simulink library "sm_flex_body_lib"  (R2016b)
settings: Solver=VariableStepAuto  StartTime=0.0  StopTime=10.0  RelTol=1e-3
values from neighbouring files (symbols this model uses):
  frameBody = splitBodyProps    [sm_flex_body_lib_fei_configure_beam.m]
undefined symbols (not defined in the file or in its folder): frameGraphic, X, Y, Z
undefined symbols (not defined in the file): beam_color, beam_opacity, beam_wall, beam_width, beamLink, brot_beamx, brot_beamy, brot_beamz, btra_beamx, elem_length, Extr_Data_Box, krot_beamx, krot_beamy, krot_beamz, ktra_beamx, rho, tau
libraries: sm_flex_body_lib x26, sm_lib x25, nesl_utility x24
(part 1 of 2)
Description:
  | Simscape Multibody Flexible Body Library v3.2
  | Copyright 2017 The MathWorks, Inc.
settings Model: Creator=smiller  LastModifiedBy=smiller

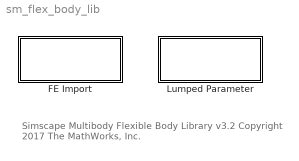
== system sm_flex_body_lib ==
  note: Simscape Multibody Flexible Body Library v3.2
      | Copyright 2017 The MathWorks, Inc.
  FE Import : Subsystem
  Lumped Parameter : Subsystem

== system sm_flex_body_lib/FE Import ==
  Bodies : Subsystem

== system sm_flex_body_lib/Lumped Parameter ==
  Bodies : Subsystem

== system sm_flex_body_lib/FE Import/Bodies ==
  Body 3 Frames : Subsystem  mask(Flexible Body via FE Import, 3 Frames){popup_massdistr=Per Interface Frame, mass=beamLink.iner.mass, com=beamLink.iner.com, moi=beamLink.iner.moi, poi=beamLink.iner.poi, splitBodyProps=beamLink.splitBodyProps(2).props, smallInertiaDim=1e-3, smallInertiaMass=1e-6, rigid_body_filename='BeamLink.stl', rigid_body_color=[0.0 0.4 0.6], rigid_body_opacity=0, intf_body_color=[0.0 0.4 0.6], intf_body_opacity=1, intf_graphic_color=[0.0 0.4 0.6], intf_graphic_opacity=0, rigidBodyFrame=2, T=beamLink.models(5).T, numframes=3, K=beamLink.models(5).K, M=beamLink.models(5).M, ksi=0.05, dofIdxMap=beamLink.models(5).dofIdxMap, tau=1e-6, H=beamLink.models(5).H, sensedFeaDofs_UI=[], numDynModes=20}
      mask prompts: popup_massdistr "Body Mass Distribution"; mass "Mass (kg)"; com "Center of Mass [xyz] (m)"; moi "Moments of Inertia (kg*m^2)"; poi "Products of Inertia (kg*m^2)"; splitBodyProps "Properties (structure)"; smallInertiaDim "Cube Side Length (m)"; smallInertiaMass "Cube Mass (kg)"; rigid_body_filename "Rigid Body File Name"; rigidBodyFrame "Rigid Body Frame"; T "Interface Frame Locations (m)"; K "Stiffness Matrix"; M "Mass Matrix"; ksi "Modal Damping Parameter"; dofIdxMap "Frame Dof Indices"; tau "Filter Time Constant (s)"; H "C-B Transformation Matrix"; sensedFeaDofs_UI "C-B Transformation Matrix Indices for Logging"
      mask help: Models a flexible body using a deflection model that relies on data imported from finite element software. Body deflection is superimposed on rigid body motion. The mass of the body can be assigned to the rigid body or distributed across each interface frame.
      mask init:
      | % Configure rigid and interface solids
      | [Nf, frameBody, frameGraphic] = sm_flex_body_lib_fei_configure_beam(gcb,splitBodyProps);
      | 
      | set_param(gcb,'numframes',num2str(Nf));
      | if(size(K,1)>0)
      |     set_param(gcb,'numDynModes',num2str(size(K,1)-Nf*6));
      | else
      |     set_param(gcb,'numDynModes','-');
      | end
      | 
      | % Sensed FEA dofs
      | if(isempty(sensedFeaDofs_UI))
      |     sensedFeaDofs = 1;
      | else
      |     sensedFeaDofs = sensedFeaDofs_UI;
      | end
      | 
      | % Create flexibility state-space model
      | [M2, L2, K2, H2] = sm_flex_body_lib_fei_form_def_matrices( ...
      |     H, M, K, ksi, Nf, dofIdxMap, rigidBodyFrame, sensedFeaDofs);
      | sys = sm_flex_body_lib_fei_form_statespace(Nf, M2, L2, K2, H2);
      | 
      | % Indices for Selector blocks at state-space output
      | sys_out_inds_frames = [1:Nf*6];
      | sys_out_width = length(sys_out_inds_frames)+length(sensedFeaDofs);
      | sys_out_inds_logging = [sys_out_width-length(sensedFeaDofs)+1:sys_out_width];
      settings: AttributesFormatString=|
      | Mass: %<popup_massdistr>
      | Interface Frames: %<numframes>
      | Rigid Frame: %<rigidBodyFrame>
      | # Dynamic Modes: %<numDynModes>
      mask Help: web('sm_flex_body_lib_fe_import_body.html');
      mask TypeOptions popup_massdistr: Single | Per Interface Frame
      mask Callback popup_massdistr:
      | maskObj = Simulink.Mask.get(gcb);
      | sms_h = maskObj.getDialogControl('cont_singlemass');
      | pms_h = maskObj.getDialogControl('cont_piecesmass');
      | int_h = maskObj.getDialogControl('cont_intfmass');
      | if strcmp(get_param(gcb,'popup_massdistr'),'Single')
      |     sms_h.Visible = 'on';
      |     int_h.Visible = 'on';
      |     pms_h.Visible = 'off';
      | else
      |     sms_h.Visible = 'off';
      |     int_h.Visible = 'off';
      |     pms_h.Visible = 'on';
      | end
      | clear maskObj sms_h pms_h int_h
      mask TypeOptions rigidBodyFrame: 1 | 2 | 3
      mask DialogControl cont_singlemass Prompt: Single Mass
      mask DialogControl cont_piecesmass Prompt: Body Mass Per Interface Frame
      mask DialogControl cont_intfmass Prompt: Interface Frame Minimum Mass
      mask DialogControl Control3 Prompt: Color [RGB]
      mask DialogControl Control4 Prompt: Opacity (0-1)
      mask DialogControl Control5 Prompt: Rigid Body Solid
      mask DialogControl Control6 Prompt: Interface Solid
      mask DialogControl Control7 Prompt: Interface Graphic
      mask Display: image('sm_flex_body_lib_feibeam3fr_IMAGE.png')
  Body 5 Frames : Subsystem  mask(Flexible Beam via FE Import, 5 Frames){popup_massdistr=Per Interface Frame, mass=beamLink.iner.mass, com=beamLink.iner.com, moi=beamLink.iner.moi, poi=beamLink.iner.poi, splitBodyProps=beamLink.splitBodyProps(3).props, smallInertiaDim=1e-3, smallInertiaMass=1e-6, rigid_body_filename='BeamLink.stl', rigid_body_color=[0.0 0.4 0.6], rigid_body_opacity=0, intf_body_color=[0.0 0.4 0.6], intf_body_opacity=1, intf_graphic_color=[0.0 0.4 0.6], intf_graphic_opacity=0, rigidBodyFrame=3, T=beamLink.models(7).T, numframes=5, K=beamLink.models(7).K, M=beamLink.models(7).M, ksi=0.05, dofIdxMap=beamLink.models(7).dofIdxMap, tau=1e-6, H=beamLink.models(7).H, sensedFeaDofs_UI=[], numDynModes=20}
      mask prompts: popup_massdistr "Body Mass Distribution"; mass "Mass (kg)"; com "Center of Mass [xyz] (m)"; moi "Moments of Inertia (kg*m^2)"; poi "Products of Inertia (kg*m^2)"; splitBodyProps "Properties (structure)"; smallInertiaDim "Cube Side Length (m)"; smallInertiaMass "Cube Mass (kg)"; rigid_body_filename "Rigid Body File Name"; rigidBodyFrame "Rigid Body Frame"; T "Interface Frame Locations (m)"; K "Stiffness Matrix"; M "Mass Matrix"; ksi "Modal Damping Parameter"; dofIdxMap "Frame Dof Indices"; tau "Filter Time Constant (s)"; H "C-B Transformation Matrix"; sensedFeaDofs_UI "C-B Transformation Matrix Indices for Logging"
      mask help: Models a flexible body using a deflection model that relies on data imported from finite element software. Body deflection is superimposed on rigid body motion. The mass of the body can be assigned to the rigid body or distributed across each interface frame.
      mask init: same as sm_flex_body_lib/FE Import/Bodies/Body 3 Frames
      settings: AttributesFormatString=|
      | Mass: %<popup_massdistr>
      | Interface Frames: %<numframes>
      | Rigid Frame: %<rigidBodyFrame>
      | # Dynamic Modes: %<numDynModes>
      mask Help: web('sm_flex_body_lib_fe_import_body.html');
      mask TypeOptions popup_massdistr: Single | Per Interface Frame
      mask Callback popup_massdistr:
      | maskObj = Simulink.Mask.get(gcb);
      | sms_h = maskObj.getDialogControl('cont_singlemass');
      | pms_h = maskObj.getDialogControl('cont_piecesmass');
      | int_h = maskObj.getDialogControl('cont_intfmass');
      | if strcmp(get_param(gcb,'popup_massdistr'),'Single')
      |     sms_h.Visible = 'on';
      |     int_h.Visible = 'on';
      |     pms_h.Visible = 'off';
      | else
      |     sms_h.Visible = 'off';
      |     int_h.Visible = 'off';
      |     pms_h.Visible = 'on';
      | end
      | clear maskObj sms_h pms_h int_h
      mask TypeOptions rigidBodyFrame: 1 | 2 | 3 | 4 | 5
      mask DialogControl cont_singlemass Prompt: Single Mass
      mask DialogControl cont_piecesmass Prompt: Body Mass Per Interface Frame
      mask DialogControl cont_intfmass Prompt: Interface Frame Minimum Mass
      mask DialogControl Control3 Prompt: Color [RGB]
      mask DialogControl Control4 Prompt: Opacity (0-1)
      mask DialogControl Control5 Prompt: Rigid Body Solid
      mask DialogControl Control6 Prompt: Interface Solid
      mask DialogControl Control7 Prompt: Interface Graphic
      mask Display: image('sm_flex_body_lib_feibeam5fr_IMAGE.png')
  Frame 1 : Subsystem  Variant=on  VariantControl=Variant1  OverrideUsingVariant=Flex
      settings: AttributesFormatString=%<ActiveVariant>
      mask Display:
      | blk = find_system(gcbh, 'SearchDepth', 1,'FollowLinks','on','LookUnderMasks','all', 'Parent', gcb, 'VariantObject', get_param(gcb,'activevariant'));
      | eval(get_param(blk, 'MaskDisplay'));
  Inertia F1 : Subsystem  mask(Flexibe Beam Frame Inertia and Graphic){frameSolid_elem=0, frameGraphic_elem=0, popup_graphicShape=Sphere, frameGraphicSize=10}
      mask prompts: frameSolid_elem "Frame Solid Data (structure)"; frameGraphic_elem "Frame Graphic Data (structure)"; popup_graphicShape "Frame Graphic Shape"; frameGraphicSize "Frame Graphic Size (pixels)"
      mask help: Models inertia at interface frame. A graphical element to display the location and orientation of the frame can also be shown.
      mask init:
      | set_param([gcb '/Deflection Graphic'],'MarkerShape',get_param(gcb,'popup_graphicShape'));
      mask TypeOptions popup_graphicShape: Sphere | Cube | Frame

== system sm_flex_body_lib/Lumped Parameter/Bodies ==
  Bearing Joint : sm_lib/Joints/Bearing Joint  SenseConstraintForce=off  SenseConstraintForceX=off  SenseConstraintForceY=off  SenseConstraintForceZ=off  SenseConstraintTorque=off  SenseConstraintTorqueX=off  SenseConstraintTorqueY=off  SenseConstraintTorqueZ=off  SenseTotalForce=off  SenseTotalForceX=off  SenseTotalForceY=off  SenseTotalForceZ=off  SenseTotalTorque=off  SenseTotalTorqueX=off  SenseTotalTorqueY=off  SenseTotalTorqueZ=off  CompositeWrenchDir=FollowerOnBase  CompositeWrenchFrame=BaseFrame  PzEquilibriumPosition=0  PzEquilibriumPositionUnits=m  PzSpringStiffness=ktra_beamx_elem  PzSpringStiffnessUnits=N/m  PzDampingCoefficient=btra_beamx_elem  PzDampingCoefficientUnits=N/(m/s)  PzTorqueActuationMode=NoTorque  PzMotionActuationMode=ComputedMotion  PzSensePosition=off  PzSenseVelocity=off  PzSenseAcceleration=off  PzSenseTorqueForce=off  PzPositionTargetSpecify=off  PzPositionTargetPriority=High  PzPositionTargetValue=0  PzPositionTargetValueUnits=m  PzVelocityTargetSpecify=off  PzVelocityTargetPriority=High  PzVelocityTargetValue=0  PzVelocityTargetValueUnits=m/s  RxEquilibriumPosition=0  RxEquilibriumPositionUnits=deg  RxSpringStiffness=krot_beamz_elem  RxSpringStiffnessUnits=N*m/rad  RxDampingCoefficient=brot_beamz_elem  RxDampingCoefficientUnits=N*m/(rad/s)  RxTorqueActuationMode=NoTorque  RxMotionActuationMode=ComputedMotion  RxSensePosition=off  RxSenseVelocity=off  RxSenseAcceleration=off  RxSenseTorqueForce=off  RxPositionTargetSpecify=off  RxPositionTargetPriority=High  RxPositionTargetValue=0  RxPositionTargetValueUnits=deg  RxVelocityTargetSpecify=off  RxVelocityTargetPriority=High  RxVelocityTargetValue=0  RxVelocityTargetValueUnits=deg/s  RyEquilibriumPosition=0  RyEquilibriumPositionUnits=deg  RySpringStiffness=krot_beamy_elem  RySpringStiffnessUnits=N*m/rad  RyDampingCoefficient=brot_beamy_elem  RyDampingCoefficientUnits=N*m/(rad/s)  RyTorqueActuationMode=NoTorque  RyMotionActuationMode=ComputedMotion  RySensePosition=off  RySenseVelocity=off  RySenseAcceleration=off  RySenseTorqueForce=off  RyPositionTargetSpecify=off  RyPositionTargetPriority=High  RyPositionTargetValue=0  RyPositionTargetValueUnits=deg  RyVelocityTargetSpecify=off  RyVelocityTargetPriority=High  RyVelocityTargetValue=0  RyVelocityTargetValueUnits=deg/s  RzEquilibriumPosition=0  RzEquilibriumPositionUnits=deg  RzSpringStiffness=krot_beamx_elem  RzSpringStiffnessUnits=N*m/rad  RzDampingCoefficient=brot_beamx_elem  RzDampingCoefficientUnits=N*m/(rad/s)  RzTorqueActuationMode=NoTorque  RzMotionActuationMode=ComputedMotion  RzSensePosition=off  RzSenseVelocity=off  RzSenseAcceleration=off  RzSenseTorqueForce=off  RzPositionTargetSpecify=off  RzPositionTargetPriority=High  RzPositionTargetValue=0  RzPositionTargetValueUnits=deg  RzVelocityTargetSpecify=off  RzVelocityTargetPriority=High  RzVelocityTargetValue=0  RzVelocityTargetValueUnits=deg/s
  Flex_Element : Subsystem  mask(Flexible Beam Element){be_length=elem_length, rho=rho, be_color=beam_color, be_opacity=beam_opacity, krot_beamz_elem=krot_beamz, brot_beamz_elem=brot_beamz, krot_beamy_elem=krot_beamy, brot_beamy_elem=brot_beamy, krot_beamx_elem=krot_beamx, brot_beamx_elem=brot_beamx, ktra_beamx_elem=ktra_beamx, btra_beamx_elem=btra_beamx, radio_flextype_elem=Rotation: Z}
      mask prompts: be_length "Beam Length (m)"; rho "Material Density (kg/(m^3))"; be_color "Color [RGB]"; be_opacity "Opacity (0-1)"; radio_flextype_elem "Flexible Element Degrees of Freedom"
      mask help: Models a flexible beam element as used in the lumped parameter method. Contains two solids connected by a joint defining the bending degrees of freedom. Select the degrees of freedom via parameters in the dialog box. The same damping coefficient is used for all degrees of freedom.
      mask init:
      | sm_flex_body_lib_lpar_configure_flextype(gcb,radio_flextype_elem)
      settings: CopyFcn=%set_param(gcb, 'LinkStatus', 'none')
      mask TypeOptions radio_flextype_elem: Rotation: Z | Rotation: X, Y, Z; Translation: X
      mask DialogControl text_k Prompt: Stiffness (N/m, Nm/rad)
      mask DialogControl text_b Prompt: Damp. (Ns/m, Nms/rad)
      mask DialogControl Control5 Prompt: About Beam Z
      mask DialogControl Control6 Prompt: About Beam Y
      mask DialogControl Control7 Prompt: About Beam X
      mask DialogControl Control8 Prompt: Along X
  Flexible Beam : Subsystem  Tag=PublishSubsystem  mask(Flexible Body, Lumped Parameter){popup_material=Steel, rho_cust=2800, youngsM_cust=7.0e+10, shearM_cust=2.6316e+10, rho_std=7.800e+03, youngsM_std=2.000e+11, shearM_std=7.720e+10, edf_beam=2.5807e-05, sdf_beam=3.2259e-06, checkbox_internalvalues=off, popup_xc=Custom, beam_width=0.015, beam_width_in=0, beam_height=0.005, beam_height_in=0, circle_diameter=0.015, circle_diameter_in=0, custom_ixx=2.6121e-003, custom_iyy=2.6121e-003, custom_ip=5.2242e-003, custom_j=1.5625e-09, extrusion_data_custom=[0.015 0.005;-0.015 0.005;-0.015 -0.005;0.015 -0.005]/2, beam_length=0.30, elem_length=0.03, numelem=10, extrusion_data=Extr_Data_Box(beam_width,beam_width-2*beam_wall,beam_width,beam_width-2*beam_wall), beam_color=[0.5 0.5 0.5], beam_opacity=1, radio_flextype=Rotation: Z}
      mask prompts: checkbox_internalvalues "Print internal values to Command Window"; popup_xc "Cross-Section Type"; custom_ixx "Area Ixx"; custom_iyy "Area Iyy"; custom_ip "Polar Ip"; custom_j "Torsion J (m^4)"; extrusion_data_custom "Extrusion data [x;y] (m)"; beam_length "Length (m)"; numelem "Number of elements"; beam_color "Color [RGB]"; beam_opacity "Opacity (0-1)"; radio_flextype "Flexible Element Degrees of Freedom"
      mask help: Models a flexible beam based on lumped parameter method. Number of flexible elements, material properties as well as beam cross section and dimensions can be varied from mask parameters.
      mask init:
      | cur_blk = gcb;
      | 
      | if(popup_xc==1)
      |     extrusion_data = Extr_Data_Box(beam_width,beam_width_in,beam_height,beam_height_in);
      |     xc_props = [beam_width beam_width_in beam_height beam_height_in];
      | elseif(popup_xc==2)
      |     extrusion_data = Extr_Data_Ring(circle_diameter/2,circle_diameter_in/2,0,360);
      |     xc_props = [circle_diameter circle_diameter_in];
      | elseif(popup_xc==3)
      |     extrusion_data = extrusion_data_custom;
      |     extrusion_data_vec = reshape(extrusion_data,[length(extrusion_data)*2,1]);
      |     xc_props = [custom_ixx;custom_iyy;custom_ip;custom_j;extrusion_data_vec];
      | end
      | 
      | if(popup_material == 1)
      |     rho = rho_cust;
      |     youngsM = youngsM_cust;
      |     shearM = shearM_cust;
      | else
      |     rho = rho_std;
      |     youngsM = youngsM_std;
      |     shearM = shearM_std;
      | end
      | 
      | 
      | [krot_beamz, krot_beamy, krot_beamx, ktra_beamx,...
      |     brot_beamz, brot_beamy, brot_beamx, btra_beamx, ...
      |     elem_length, Ixx, Iyy, J, crossArea] = ...
      |     sm_flex_body_lib_lpar_compute_flexprop(youngsM, shearM, numelem, beam_length, ...
      |     edf_beam, sdf_beam,popup_xc, xc_props);
      | 
      | if(checkbox_internalvalues)
      |     temp_intvaltable = table(...
      |         [Ixx;Iyy;J;crossArea;elem_length;...
      |         krot_beamz;krot_beamy;krot_beamx;ktra_beamx;...
      |         brot_beamz;brot_beamy;brot_beamx;btra_beamx],...
      |         {'m^4';'m^4';'m^4';'m^2';'m';...
      |         'N*m/rad';'N*m/rad';'N*m/rad';'N/m';...
      |         'N*m/(rad/s)';'N*m/(rad/s)';'N*m/(rad/s)';'N/(m/s)'},...
      |         'VariableNames',{'Value','Units'},'RowNames',...
      |         {'Area Moment of Inertia, Ixx','Area Moment of Inertia, Iyy',...
      |         'Torsional Constant, J','Cross sectional area, A','Flexible element length',...
      |         'Element Stiffness, Bending about Z','Element Stiffness, Bending about Y',...
      |         'Element Stiffness, Torsion about X','Element Stiffness, Elongation along X',...
      |         'Element Damping, Bending about Z','Element Damping, Bending about Y',...
      |         'Element Damping, Torsion about X','Element Damping, Elongation along X'});
      |     disp(temp_intvaltable);
      | end
      | 
      | set_param(cur_blk,'elem_length',num2str(elem_length));
      | 
      | sm_flex_body_lib_lpar_construct_beam(cur_blk,numelem,get_param(cur_blk,'radio_flextype'));
      | 
      | clear xc_props
      settings: CopyFcn=%set_param(gcb, 'LinkStatus', 'none')
      settings: AttributesFormatString=|
      | No of Elem: 10
      | Rotation: Z
      mask Help: web('sm_flex_body_lib_lumped_par_beam.html')
      mask TypeOptions popup_material: Custom | Steel | Aluminum | Brass | Bismuth | Copper | Gold | Iron | Lead | Magnesium | Nickel | Silver | Tin | Zinc
      mask Callback popup_material:
      | maskObj = Simulink.Mask.get(gcb);
      | contcm_h = maskObj.getDialogControl('cont_custmaterial');
      | contsm_h = maskObj.getDialogControl('cont_stdmaterial');
      | 
      | rhostd_h = maskObj.getParameter('rho_std');
      | youngM_h = maskObj.getParameter('youngsM_std');
      | shearM_h = maskObj.getParameter('shearM_std');
      | 
      | popup_cm = get_param(gcb,'popup_material');
      | if strcmp(popup_cm,'Custom')
      |     contcm_h.Visible = 'on';
      |     contsm_h.Visible = 'off';
      | else
      |     [rho, E, G] = sm_flex_body_lib_lpar_matprops(popup_cm);
      |     rhostd_h.ReadOnly = 'off';
      |     youngM_h.ReadOnly = 'off';
      |     shearM_h.ReadOnly = 'off';
      |     set_param(gcb,'rho_std',sprintf('%0.3e',rho));
      |     set_param(gcb,'youngsM_std',sprintf('%0.3e',E));
      |     set_param(gcb,'shearM_std',sprintf('%0.3e',G));
      | 	rhostd_h.ReadOnly = 'on';
      |     youngM_h.ReadOnly = 'on';
      |     shearM_h.ReadOnly = 'on';
      |     contcm_h.Visible = 'off';
      |     contsm_h.Visible = 'on';
      | end
      | 
      | clear maskObj contcm_h contsm_h
      | clear rhostd_h youngM_h shearM_h rho E G
      mask TypeOptions popup_xc: Hollow Rectangle | Hollow Circle | Custom
      mask Callback popup_xc:
      | maskObj = Simulink.Mask.get(gcb);
      | rcti_h = maskObj.getDialogControl('container_rectimage');
      | rctp_h = maskObj.getDialogControl('container_rectparams');
      | ciri_h = maskObj.getDialogControl('container_circleimage');
      | cirp_h = maskObj.getDialogControl('container_circleparams');
      | cusi_h = maskObj.getDialogControl('container_customimage');
      | cusp_h = maskObj.getDialogControl('container_customparams');
      | 
      | popd_h = maskObj.getParameter('popup_dampparam');
      | contdr_h = maskObj.getDialogControl('cont_dampingratio');
      | contdc_h = maskObj.getDialogControl('cont_dampingcoeff');
      | 
      | rcti_h.Visible = 'off';
      | rctp_h.Visible = 'off';
      | ciri_h.Visible = 'off';
      | cirp_h.Visible = 'off';
      | cusi_h.Visible = 'off';
      | cusp_h.Visible = 'off';
      | 
      | if strcmp(get_param(gcb,'popup_xc'),'Hollow Rectangle')
      |     rcti_h.Visible = 'on';
      |     rctp_h.Visible = 'on';
      | elseif strcmp(get_param(gcb,'popup_xc'),'Hollow Circle')
      |     ciri_h.Visible = 'on';
      |     cirp_h.Visible = 'on';
      | elseif strcmp(get_param(gcb,'popup_xc'),'Custom')
      |     cusi_h.Visible = 'on';
      |     cusp_h.Visible = 'on';
      | end
      | 
      | clear rcti_h rctp_h ciri_h cirp_h cusi_h cusp_h
      mask TypeOptions radio_flextype: Rotation: Z | Rotation: X, Y, Z; Translation: X
      mask DialogControl Control20 Prompt: Material
      mask DialogControl grp_damping Prompt: Damping
      mask DialogControl text_outer Prompt: Outer
      mask DialogControl text_inner Prompt: Inner
      mask DialogControl text_width Prompt: Width (m)
      mask DialogControl text_height Prompt: Height (m)
      mask DialogControl text_circle_outer Prompt: Outer
      mask DialogControl text_circle_inner Prompt: Inner
      mask DialogControl text_circle_width Prompt: Diameter (m)
      mask DialogControl cont_custmoi Prompt: Moment of Inertia (m^4)
      mask Display: image('sm_flex_body_lib_lumpparbeam_IMAGE.png');
  Revolute Joint : sm_lib/Joints/Revolute Joint  SenseConstraintForce=off  SenseConstraintForceX=off  SenseConstraintForceY=off  SenseConstraintForceZ=off  SenseConstraintTorque=off  SenseConstraintTorqueX=off  SenseConstraintTorqueY=off  SenseConstraintTorqueZ=off  SenseTotalForce=off  SenseTotalForceX=off  SenseTotalForceY=off  SenseTotalForceZ=off  SenseTotalTorque=off  SenseTotalTorqueX=off  SenseTotalTorqueY=off  SenseTotalTorqueZ=off  CompositeWrenchDir=FollowerOnBase  CompositeWrenchFrame=BaseFrame  EquilibriumPosition=0  EquilibriumPositionUnits=deg  SpringStiffness=krot_beamz_elem  SpringStiffnessUnits=N*m/rad  DampingCoefficient=brot_beamz_elem  DampingCoefficientUnits=N*m/(rad/s)  TorqueActuationMode=NoTorque  MotionActuationMode=ComputedMotion  SensePosition=off  SenseVelocity=off  SenseAcceleration=off  SenseTorqueForce=off  PositionTargetSpecify=off  PositionTargetPriority=High  PositionTargetValue=0  PositionTargetValueUnits=deg  VelocityTargetSpecify=off  VelocityTargetPriority=High  VelocityTargetValue=0  VelocityTargetValueUnits=deg/s

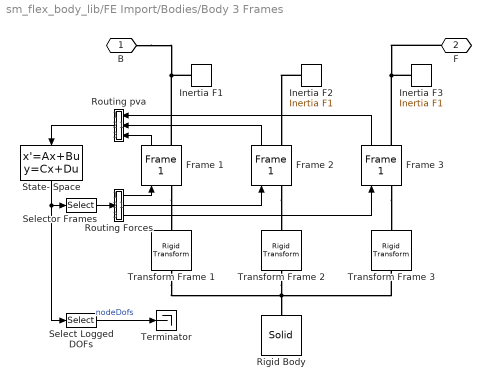
== system sm_flex_body_lib/FE Import/Bodies/Body 3 Frames ==
  Frame 1 : sm_flex_body_lib/FE Import/Bodies/Frame 1  SystemSampleTime=-1  VariantControl=Variant1  OverrideUsingVariant=Flex
      settings: AttributesFormatString=%<ActiveVariant>
  Frame 2 : sm_flex_body_lib/FE Import/Bodies/Frame 1  SystemSampleTime=-1  VariantControl=Variant1  OverrideUsingVariant=Rigid
      settings: AttributesFormatString=%<ActiveVariant>
  Frame 3 : sm_flex_body_lib/FE Import/Bodies/Frame 1  SystemSampleTime=-1  VariantControl=Variant1  OverrideUsingVariant=Flex
      settings: AttributesFormatString=%<ActiveVariant>
  Inertia F1 : sm_flex_body_lib/FE Import/Bodies/Inertia F1  frameSolid_elem=frameBody(1)  frameGraphic_elem=frameGraphic(1)  popup_graphicShape=Sphere  frameGraphicSize=10
  Inertia F2 : sm_flex_body_lib/FE Import/Bodies/Inertia F1  frameSolid_elem=frameBody(2)  frameGraphic_elem=frameGraphic(2)  popup_graphicShape=Sphere  frameGraphicSize=10
  Inertia F3 : sm_flex_body_lib/FE Import/Bodies/Inertia F1  frameSolid_elem=frameBody(3)  frameGraphic_elem=frameGraphic(3)  popup_graphicShape=Sphere  frameGraphicSize=10
  Rigid Body : sm_lib/Body Elements/Solid  InertiaType=Custom  Mass=0  MassUnits=kg  CenterOfMass=[0 0 0]  CenterOfMassUnits=m  MomentsOfInertia=[0 0 0]  MomentsOfInertiaUnits=kg*m^2  ProductsOfInertia=[0 0 0]  ProductsOfInertiaUnits=kg*m^2  DensityBased=on  Density=1000  DensityUnits=kg/m^3  DoExposeReferenceFrame=on  SerializedFrames=<Frames/>  GraphicType=FromGeometry  MarkerShape=Sphere  MarkerSize=10  GraphicVisPropType=SimpleVisualProperties  GraphicDiffuseColor=rigid_body_color  GraphicSpecularColor=[0.5 0.5 0.5 1.0]  GraphicAmbientColor=[0.15 0.15 0.15 1.0]  GraphicEmissiveColor=[0.0 0.0 0.0 1.0]  GraphicShininess=75  GraphicOpacity=rigid_body_opacity  GeometryShape=FromFile  RectangleSize=[1 1]  RectangleSizeUnits=m  BrickDimensions=[1 1 1]  BrickDimensionUnits=m  CylinderRadius=1  CylinderRadiusUnits=m  CylinderLength=1  CylinderLengthUnits=m  SphereRadius=1  SphereRadiusUnits=m  EllipsoidRadii=[1 1 1]  EllipsoidRadiiUnits=m  ExtrusionCrossSection=[1 1; -1 1; -1 -1; 1 -1]  ExtrusionCrossSectionUnits=m  ExtrusionLength=1  ExtrusionLengthUnits=m  PolygonNumSides=3  PolygonOuterRadius=1  PolygonOuterRadiusUnits=m  ExtGeomFileType=STL  ExtGeomFileName=BeamLink.stl  ExtGeomFileUnits=m  RevolutionCrossSection=[1 1; 1 -1; 2 -1; 2 1]  RevolutionCrossSectionUnits=m  RevolutionExtent=Full  RevolutionAngle=180  RevolutionAngleUnits=deg
  Routing Forces : Subsystem
  Routing pva : Subsystem
  Select Logged DOFs : Selector  InputPortWidth=sys_out_width  IndexOptions=Index vector (dialog)  Indices=sys_out_inds_logging  OutputSizes=1
  Selector Frames : Selector  InputPortWidth=sys_out_width  IndexOptions=Index vector (dialog)  Indices=sys_out_inds_frames  OutputSizes=1
  State- Space : StateSpace  A=sys.A  B=sys.B  C=sys.C  D=sys.D  X0=0
  Terminator : Terminator
  Transform Frame 1 : sm_lib/Frames and Transforms/Rigid Transform  TranslationMethod=Cartesian  TranslationStandardOffset=0  TranslationLengthUnit=m  TranslationStandardAxis=+Z  TranslationCartesianOffset=T(1,:)  TranslationROffset=0  TranslationROffsetUnits=m  TranslationZOffset=0  TranslationZOffsetUnits=m  TranslationThetaOffset=0  TranslationThetaOffsetUnits=deg  RotationMethod=None  RotationAngleUnits=deg  RotationStandardAxis=+Z  RotationAngle=0.0  RotationArbitraryAxis=[0 0 1]  FollAlignAxisA=+X  BaseAlignAxisA=+Y  FollAlignAxisB=+Y  BaseAlignAxisB=+Z  RotationSequenceAxes=FollowerAxes  RotationSequence=XYX  RotationSequenceAngles=[0 0 0]  RotationSequenceAnglesUnits=deg  RotationMatrix=[1 0 0; 0 1 0; 0 0 1]
  Transform Frame 2 : sm_lib/Frames and Transforms/Rigid Transform  TranslationMethod=Cartesian  TranslationStandardOffset=0  TranslationLengthUnit=m  TranslationStandardAxis=+Z  TranslationCartesianOffset=T(2,:)  TranslationROffset=0  TranslationROffsetUnits=m  TranslationZOffset=0  TranslationZOffsetUnits=m  TranslationThetaOffset=0  TranslationThetaOffsetUnits=deg  RotationMethod=None  RotationAngleUnits=deg  RotationStandardAxis=+Z  RotationAngle=0.0  RotationArbitraryAxis=[0 0 1]  FollAlignAxisA=+X  BaseAlignAxisA=+Y  FollAlignAxisB=+Y  BaseAlignAxisB=+Z  RotationSequenceAxes=FollowerAxes  RotationSequence=XYX  RotationSequenceAngles=[0 0 0]  RotationSequenceAnglesUnits=deg  RotationMatrix=[1 0 0; 0 1 0; 0 0 1]
  Transform Frame 3 : sm_lib/Frames and Transforms/Rigid Transform  TranslationMethod=Cartesian  TranslationStandardOffset=0  TranslationLengthUnit=m  TranslationStandardAxis=+Z  TranslationCartesianOffset=T(3,:)  TranslationROffset=0  TranslationROffsetUnits=m  TranslationZOffset=0  TranslationZOffsetUnits=m  TranslationThetaOffset=0  TranslationThetaOffsetUnits=deg  RotationMethod=None  RotationAngleUnits=deg  RotationStandardAxis=+Z  RotationAngle=0.0  RotationArbitraryAxis=[0 0 1]  FollAlignAxisA=+X  BaseAlignAxisA=+Y  FollAlignAxisB=+Y  BaseAlignAxisB=+Z  RotationSequenceAxes=FollowerAxes  RotationSequence=XYX  RotationSequenceAngles=[0 0 0]  RotationSequenceAnglesUnits=deg  RotationMatrix=[1 0 0; 0 1 0; 0 0 1]
  B : PMIOPort  Port=1  Side=Left
  F : PMIOPort  Port=2  Side=Right
  wires:
  Frame 3/1 -> Routing pva/1(p3)
  Routing Forces/3(F3) -> Frame 3/1
  Frame 2/1 -> Routing pva/2(p2)
  Routing Forces/2(F2) -> Frame 2/1
  Routing Forces/1(F1) -> Frame 1/1
  Routing pva/1(Out1) -> State- Space/1
  Frame 1/1 -> Routing pva/3(p1)
  Select Logged DOFs/1 -> Terminator/1  "nodeDofs"
  Selector Frames/1 -> Routing Forces/1(In1)
  State- Space/1 -> Select Logged DOFs/1, Selector Frames/1
  connections:
  Frame 3/LConn1 -- Transform Frame 3/RConn1
  Frame 3/RConn1 -- Inertia F3/LConn1 -- F/RConn1
  Frame 2/LConn1 -- Transform Frame 2/RConn1
  Frame 1/LConn1 -- Transform Frame 1/RConn1
  Inertia F2/LConn1 -- Frame 2/RConn1
  Transform Frame 3/LConn1 -- Transform Frame 2/LConn1 -- Rigid Body/RConn1 -- Transform Frame 1/LConn1
  B/RConn1 -- Inertia F1/LConn1 -- Frame 1/RConn1

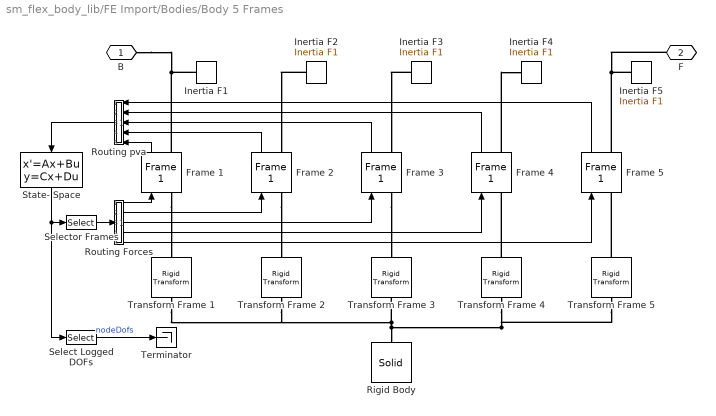
== system sm_flex_body_lib/FE Import/Bodies/Body 5 Frames ==
  Frame {1..2,4..5} (4 alike) : sm_flex_body_lib/FE Import/Bodies/Frame 1  SystemSampleTime=-1  VariantControl=Variant1  OverrideUsingVariant=Flex
      settings: AttributesFormatString=%<ActiveVariant>
  Frame 3 : sm_flex_body_lib/FE Import/Bodies/Frame 1  SystemSampleTime=-1  VariantControl=Variant1  OverrideUsingVariant=Rigid
      settings: AttributesFormatString=%<ActiveVariant>
  Inertia F1 : sm_flex_body_lib/FE Import/Bodies/Inertia F1  frameSolid_elem=frameBody(1)  frameGraphic_elem=frameGraphic(1)  popup_graphicShape=Sphere  frameGraphicSize=10
  Inertia F2 : sm_flex_body_lib/FE Import/Bodies/Inertia F1  frameSolid_elem=frameBody(2)  frameGraphic_elem=frameGraphic(2)  popup_graphicShape=Sphere  frameGraphicSize=10
  Inertia F3 : sm_flex_body_lib/FE Import/Bodies/Inertia F1  frameSolid_elem=frameBody(3)  frameGraphic_elem=frameGraphic(3)  popup_graphicShape=Sphere  frameGraphicSize=10
  Inertia F4 : sm_flex_body_lib/FE Import/Bodies/Inertia F1  frameSolid_elem=frameBody(4)  frameGraphic_elem=frameGraphic(4)  popup_graphicShape=Sphere  frameGraphicSize=10
  Inertia F5 : sm_flex_body_lib/FE Import/Bodies/Inertia F1  frameSolid_elem=frameBody(5)  frameGraphic_elem=frameGraphic(5)  popup_graphicShape=Sphere  frameGraphicSize=10
  Rigid Body : sm_lib/Body Elements/Solid  InertiaType=Custom  Mass=0  MassUnits=kg  CenterOfMass=[0 0 0]  CenterOfMassUnits=m  MomentsOfInertia=[0 0 0]  MomentsOfInertiaUnits=kg*m^2  ProductsOfInertia=[0 0 0]  ProductsOfInertiaUnits=kg*m^2  DensityBased=on  Density=1000  DensityUnits=kg/m^3  DoExposeReferenceFrame=on  SerializedFrames=<Frames/>  GraphicType=FromGeometry  MarkerShape=Sphere  MarkerSize=10  GraphicVisPropType=SimpleVisualProperties  GraphicDiffuseColor=rigid_body_color  GraphicSpecularColor=[0.5 0.5 0.5 1.0]  GraphicAmbientColor=[0.15 0.15 0.15 1.0]  GraphicEmissiveColor=[0.0 0.0 0.0 1.0]  GraphicShininess=75  GraphicOpacity=rigid_body_opacity  GeometryShape=FromFile  RectangleSize=[1 1]  RectangleSizeUnits=m  BrickDimensions=[1 1 1]  BrickDimensionUnits=m  CylinderRadius=1  CylinderRadiusUnits=m  CylinderLength=1  CylinderLengthUnits=m  SphereRadius=1  SphereRadiusUnits=m  EllipsoidRadii=[1 1 1]  EllipsoidRadiiUnits=m  ExtrusionCrossSection=[1 1; -1 1; -1 -1; 1 -1]  ExtrusionCrossSectionUnits=m  ExtrusionLength=1  ExtrusionLengthUnits=m  PolygonNumSides=3  PolygonOuterRadius=1  PolygonOuterRadiusUnits=m  ExtGeomFileType=STL  ExtGeomFileName=BeamLink.stl  ExtGeomFileUnits=m  RevolutionCrossSection=[1 1; 1 -1; 2 -1; 2 1]  RevolutionCrossSectionUnits=m  RevolutionExtent=Full  RevolutionAngle=180  RevolutionAngleUnits=deg
  Routing Forces : Subsystem
  Routing pva : Subsystem
  Select Logged DOFs : Selector  InputPortWidth=sys_out_width  IndexOptions=Index vector (dialog)  Indices=sys_out_inds_logging  OutputSizes=1
  Selector Frames : Selector  InputPortWidth=sys_out_width  IndexOptions=Index vector (dialog)  Indices=sys_out_inds_frames  OutputSizes=1
  State- Space : StateSpace  A=sys.A  B=sys.B  C=sys.C  D=sys.D  X0=0
  Terminator : Terminator
  Transform Frame 1 : sm_lib/Frames and Transforms/Rigid Transform  TranslationMethod=Cartesian  TranslationStandardOffset=0  TranslationLengthUnit=m  TranslationStandardAxis=+Z  TranslationCartesianOffset=T(1,:)  TranslationROffset=0  TranslationROffsetUnits=m  TranslationZOffset=0  TranslationZOffsetUnits=m  TranslationThetaOffset=0  TranslationThetaOffsetUnits=deg  RotationMethod=None  RotationAngleUnits=deg  RotationStandardAxis=+Z  RotationAngle=0.0  RotationArbitraryAxis=[0 0 1]  FollAlignAxisA=+X  BaseAlignAxisA=+Y  FollAlignAxisB=+Y  BaseAlignAxisB=+Z  RotationSequenceAxes=FollowerAxes  RotationSequence=XYX  RotationSequenceAngles=[0 0 0]  RotationSequenceAnglesUnits=deg  RotationMatrix=[1 0 0; 0 1 0; 0 0 1]
  Transform Frame 2 : sm_lib/Frames and Transforms/Rigid Transform  TranslationMethod=Cartesian  TranslationStandardOffset=0  TranslationLengthUnit=m  TranslationStandardAxis=+Z  TranslationCartesianOffset=T(2,:)  TranslationROffset=0  TranslationROffsetUnits=m  TranslationZOffset=0  TranslationZOffsetUnits=m  TranslationThetaOffset=0  TranslationThetaOffsetUnits=deg  RotationMethod=None  RotationAngleUnits=deg  RotationStandardAxis=+Z  RotationAngle=0.0  RotationArbitraryAxis=[0 0 1]  FollAlignAxisA=+X  BaseAlignAxisA=+Y  FollAlignAxisB=+Y  BaseAlignAxisB=+Z  RotationSequenceAxes=FollowerAxes  RotationSequence=XYX  RotationSequenceAngles=[0 0 0]  RotationSequenceAnglesUnits=deg  RotationMatrix=[1 0 0; 0 1 0; 0 0 1]
  Transform Frame 3 : sm_lib/Frames and Transforms/Rigid Transform  TranslationMethod=Cartesian  TranslationStandardOffset=0  TranslationLengthUnit=m  TranslationStandardAxis=+Z  TranslationCartesianOffset=T(3,:)  TranslationROffset=0  TranslationROffsetUnits=m  TranslationZOffset=0  TranslationZOffsetUnits=m  TranslationThetaOffset=0  TranslationThetaOffsetUnits=deg  RotationMethod=None  RotationAngleUnits=deg  RotationStandardAxis=+Z  RotationAngle=0.0  RotationArbitraryAxis=[0 0 1]  FollAlignAxisA=+X  BaseAlignAxisA=+Y  FollAlignAxisB=+Y  BaseAlignAxisB=+Z  RotationSequenceAxes=FollowerAxes  RotationSequence=XYX  RotationSequenceAngles=[0 0 0]  RotationSequenceAnglesUnits=deg  RotationMatrix=[1 0 0; 0 1 0; 0 0 1]
  Transform Frame 4 : sm_lib/Frames and Transforms/Rigid Transform  TranslationMethod=Cartesian  TranslationStandardOffset=0  TranslationLengthUnit=m  TranslationStandardAxis=+Z  TranslationCartesianOffset=T(4,:)  TranslationROffset=0  TranslationROffsetUnits=m  TranslationZOffset=0  TranslationZOffsetUnits=m  TranslationThetaOffset=0  TranslationThetaOffsetUnits=deg  RotationMethod=None  RotationAngleUnits=deg  RotationStandardAxis=+Z  RotationAngle=0.0  RotationArbitraryAxis=[0 0 1]  FollAlignAxisA=+X  BaseAlignAxisA=+Y  FollAlignAxisB=+Y  BaseAlignAxisB=+Z  RotationSequenceAxes=FollowerAxes  RotationSequence=XYX  RotationSequenceAngles=[0 0 0]  RotationSequenceAnglesUnits=deg  RotationMatrix=[1 0 0; 0 1 0; 0 0 1]
  Transform Frame 5 : sm_lib/Frames and Transforms/Rigid Transform  TranslationMethod=Cartesian  TranslationStandardOffset=0  TranslationLengthUnit=m  TranslationStandardAxis=+Z  TranslationCartesianOffset=T(5,:)  TranslationROffset=0  TranslationROffsetUnits=m  TranslationZOffset=0  TranslationZOffsetUnits=m  TranslationThetaOffset=0  TranslationThetaOffsetUnits=deg  RotationMethod=None  RotationAngleUnits=deg  RotationStandardAxis=+Z  RotationAngle=0.0  RotationArbitraryAxis=[0 0 1]  FollAlignAxisA=+X  BaseAlignAxisA=+Y  FollAlignAxisB=+Y  BaseAlignAxisB=+Z  RotationSequenceAxes=FollowerAxes  RotationSequence=XYX  RotationSequenceAngles=[0 0 0]  RotationSequenceAnglesUnits=deg  RotationMatrix=[1 0 0; 0 1 0; 0 0 1]
  B : PMIOPort  Port=1  Side=Left
  F : PMIOPort  Port=2  Side=Right
  wires:
  Frame 1/1 -> Routing pva/5(p5)
  Routing pva/1(Out1) -> State- Space/1
  Routing Forces/1(F1) -> Frame 1/1
  Routing Forces/2(F2) -> Frame 2/1
  Frame 2/1 -> Routing pva/4(p4)
  Routing Forces/3(F3) -> Frame 3/1
  Frame 3/1 -> Routing pva/3(p1)
  Frame 5/1 -> Routing pva/1(p3)
  Frame 4/1 -> Routing pva/2(p2)
  Routing Forces/4(F4) -> Frame 4/1
  Routing Forces/5(F5) -> Frame 5/1
  State- Space/1 -> Select Logged DOFs/1, Selector Frames/1
  Selector Frames/1 -> Routing Forces/1(In1)
  Select Logged DOFs/1 -> Terminator/1  "nodeDofs"
  connections:
  Frame 1/RConn1 -- Inertia F1/LConn1 -- B/RConn1
  Rigid Body/RConn1 -- Transform Frame 5/LConn1 -- Transform Frame 4/LConn1 -- Transform Frame 1/LConn1 -- Transform Frame 2/LConn1 -- Transform Frame 3/LConn1
  Inertia F2/LConn1 -- Frame 2/RConn1
  Frame 1/LConn1 -- Transform Frame 1/RConn1
  Frame 2/LConn1 -- Transform Frame 2/RConn1
  Inertia F3/LConn1 -- Frame 3/RConn1
  Frame 3/LConn1 -- Transform Frame 3/RConn1
  Transform Frame 4/RConn1 -- Frame 4/LConn1
  F/RConn1 -- Frame 5/RConn1 -- Inertia F5/LConn1
  Frame 4/RConn1 -- Inertia F4/LConn1
  Transform Frame 5/RConn1 -- Frame 5/LConn1

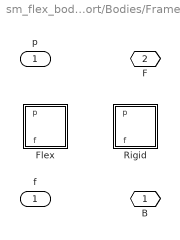
== system sm_flex_body_lib/FE Import/Bodies/Frame 1 ==
  "f " : Inport
  Flex : Subsystem  VariantControl=Flex
      mask Display: image('sm_flex_body_lib_feibeam_intfFlex_IMAGE.png');
  Rigid : Subsystem  VariantControl=Rigid
      mask Display: image('sm_flex_body_lib_feibeam_intfRigid_IMAGE.png');
  " B " : PMIOPort  Port=1  Side=Left
  " F " : PMIOPort  Port=2  Side=Right
  " p" : Outport

== system sm_flex_body_lib/FE Import/Bodies/Inertia F1 ==
  Deflection Graphic : sm_lib/Body Elements/Graphic  GraphicType=Marker  MarkerShape=Sphere  MarkerSize=frameGraphicSize  GraphicVisPropType=SimpleVisualProperties  GraphicDiffuseColor=frameGraphic_elem.color  GraphicSpecularColor=[0.5 0.5 0.5 1.0]  GraphicAmbientColor=[0.15 0.15 0.15 1.0]  GraphicEmissiveColor=[0.0 0.0 0.0 1.0]  GraphicShininess=75  GraphicOpacity=frameGraphic_elem.opacity
  Rigid Transform : sm_lib/Frames and Transforms/Rigid Transform  TranslationMethod=Cartesian  TranslationStandardOffset=0  TranslationLengthUnit=m  TranslationStandardAxis=+Z  TranslationCartesianOffset=frameSolid_elem.offset  TranslationROffset=0  TranslationROffsetUnits=m  TranslationZOffset=0  TranslationZOffsetUnits=m  TranslationThetaOffset=0  TranslationThetaOffsetUnits=deg  RotationMethod=None  RotationAngleUnits=deg  RotationStandardAxis=+Z  RotationAngle=0.0  RotationArbitraryAxis=[0 0 1]  FollAlignAxisA=+X  BaseAlignAxisA=+Y  FollAlignAxisB=+Y  BaseAlignAxisB=+Z  RotationSequenceAxes=FollowerAxes  RotationSequence=XYX  RotationSequenceAngles=[0 0 0]  RotationSequenceAnglesUnits=deg  RotationMatrix=[1 0 0; 0 1 0; 0 0 1]
  Solid : sm_lib/Body Elements/Solid  InertiaType=Custom  Mass=frameSolid_elem.mass  MassUnits=kg  CenterOfMass=frameSolid_elem.com  CenterOfMassUnits=m  MomentsOfInertia=frameSolid_elem.moi  MomentsOfInertiaUnits=kg*m^2  ProductsOfInertia=frameSolid_elem.poi  ProductsOfInertiaUnits=kg*m^2  DensityBased=off  Density=1000  DensityUnits=kg/m^3  DoExposeReferenceFrame=on  SerializedFrames=<Frames/>  GraphicType=FromGeometry  MarkerShape=Sphere  MarkerSize=10  GraphicVisPropType=SimpleVisualProperties  GraphicDiffuseColor=frameSolid_elem.color  GraphicSpecularColor=[0.5 0.5 0.5 1.0]  GraphicAmbientColor=[0.15 0.15 0.15 1.0]  GraphicEmissiveColor=[0.0 0.0 0.0 1.0]  GraphicShininess=75  GraphicOpacity=frameSolid_elem.opacity  GeometryShape=Brick  RectangleSize=[1 1]  RectangleSizeUnits=m  BrickDimensions=frameSolid_elem.dim  BrickDimensionUnits=m  CylinderRadius=1  CylinderRadiusUnits=m  CylinderLength=1  CylinderLengthUnits=m  SphereRadius=1  SphereRadiusUnits=m  EllipsoidRadii=[1 1 1]  EllipsoidRadiiUnits=m  ExtrusionCrossSection=[1 1; -1 1; -1 -1; 1 -1]  ExtrusionCrossSectionUnits=m  ExtrusionLength=1  ExtrusionLengthUnits=m  PolygonNumSides=3  PolygonOuterRadius=1  PolygonOuterRadiusUnits=m  ExtGeomFileType=STEP  ExtGeomFileUnits=m  RevolutionCrossSection=[1 1; 1 -1; 2 -1; 2 1]  RevolutionCrossSectionUnits=m  RevolutionExtent=Full  RevolutionAngle=180  RevolutionAngleUnits=deg
  B : PMIOPort  Port=1  Side=Left
  connections:
  Rigid Transform/LConn1 -- Solid/RConn1
  Deflection Graphic/RConn1 -- B/RConn1 -- Rigid Transform/RConn1

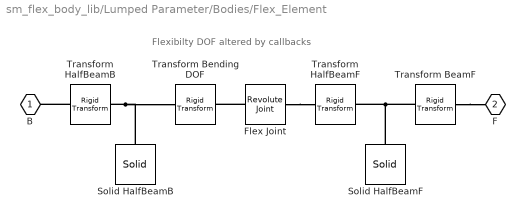
== system sm_flex_body_lib/Lumped Parameter/Bodies/Flex_Element ==
  note: Flexibilty DOF altered by callbacks
  " Transform BeamF" : sm_lib/Frames and Transforms/Rigid Transform  TranslationMethod=StandardAxis  TranslationStandardOffset=be_length/4  TranslationLengthUnit=m  TranslationStandardAxis=+Z  TranslationCartesianOffset=[0 0 0]  TranslationROffset=0  TranslationROffsetUnits=m  TranslationZOffset=0  TranslationZOffsetUnits=m  TranslationThetaOffset=0  TranslationThetaOffsetUnits=deg  RotationMethod=None  RotationAngleUnits=deg  RotationStandardAxis=+Z  RotationAngle=0  RotationArbitraryAxis=[0 0 1]  FollAlignAxisA=+X  BaseAlignAxisA=+Y  FollAlignAxisB=+Y  BaseAlignAxisB=+Z  RotationSequenceAxes=FollowerAxes  RotationSequence=XYX  RotationSequenceAngles=[0 0 0]  RotationSequenceAnglesUnits=deg  RotationMatrix=[1 0 0; 0 1 0; 0 0 1]
  Flex Joint : sm_lib/Joints/Revolute Joint  SenseConstraintForce=off  SenseConstraintForceX=off  SenseConstraintForceY=off  SenseConstraintForceZ=off  SenseConstraintTorque=off  SenseConstraintTorqueX=off  SenseConstraintTorqueY=off  SenseConstraintTorqueZ=off  SenseTotalForce=off  SenseTotalForceX=off  SenseTotalForceY=off  SenseTotalForceZ=off  SenseTotalTorque=off  SenseTotalTorqueX=off  SenseTotalTorqueY=off  SenseTotalTorqueZ=off  CompositeWrenchDir=FollowerOnBase  CompositeWrenchFrame=BaseFrame  EquilibriumPosition=0  EquilibriumPositionUnits=deg  SpringStiffness=krot_beamz_elem  SpringStiffnessUnits=N*m/rad  DampingCoefficient=brot_beamz_elem  DampingCoefficientUnits=N*m/(rad/s)  TorqueActuationMode=NoTorque  MotionActuationMode=ComputedMotion  SensePosition=off  SenseVelocity=off  SenseAcceleration=off  SenseTorqueForce=off  PositionTargetSpecify=off  PositionTargetPriority=High  PositionTargetValue=0  PositionTargetValueUnits=deg  VelocityTargetSpecify=off  VelocityTargetPriority=High  VelocityTargetValue=0  VelocityTargetValueUnits=deg/s
  Solid HalfBeamB : sm_lib/Body Elements/Solid  InertiaType=CalculateFromGeometry  Mass=1  MassUnits=kg  CenterOfMass=[0 0 0]  CenterOfMassUnits=m  MomentsOfInertia=[1 1 1]  MomentsOfInertiaUnits=kg*m^2  ProductsOfInertia=[0 0 0]  ProductsOfInertiaUnits=kg*m^2  DensityBased=on  Density=rho  DensityUnits=kg/(m^3)  DoExposeReferenceFrame=on  SerializedFrames=<Frames/>  GraphicType=FromGeometry  MarkerShape=Sphere  MarkerSize=10  MarkerSizeUnits=m  GraphicVisPropType=SimpleVisualProperties  GraphicDiffuseColor=be_color  GraphicSpecularColor=[0.5 0.5 0.5 1.0]  GraphicAmbientColor=[0.15 0.15 0.15 1.0]  GraphicEmissiveColor=[0.0 0.0 0.0 1.0]  GraphicShininess=75  GraphicOpacity=be_opacity  GeometryShape=GeneralExtrusion  RectangleSize=[1 1]  RectangleSizeUnits=m  BrickDimensions=[1 1 1]  BrickDimensionUnits=m  CylinderRadius=1  CylinderRadiusUnits=m  CylinderLength=1  CylinderLengthUnits=m  SphereRadius=1  SphereRadiusUnits=m  EllipsoidRadii=[1 1 1]  EllipsoidRadiiUnits=m  ExtrusionCrossSection=extrusion_data  ExtrusionCrossSectionUnits=m  ExtrusionLength=be_length/2  ExtrusionLengthUnits=m  PolygonNumSides=3  PolygonOuterRadius=1  PolygonOuterRadiusUnits=m  ExtGeomFileType=STL  ExtGeomFileUnits=m  RevolutionCrossSection=[1 1; 1 -1; 2 -1; 2 1]  RevolutionCrossSectionUnits=m  RevolutionExtent=Full  RevolutionAngle=180  RevolutionAngleUnits=deg
  Solid HalfBeamF : sm_lib/Body Elements/Solid  InertiaType=CalculateFromGeometry  Mass=1  MassUnits=kg  CenterOfMass=[0 0 0]  CenterOfMassUnits=m  MomentsOfInertia=[1 1 1]  MomentsOfInertiaUnits=kg*m^2  ProductsOfInertia=[0 0 0]  ProductsOfInertiaUnits=kg*m^2  DensityBased=on  Density=rho  DensityUnits=kg/(m^3)  DoExposeReferenceFrame=on  SerializedFrames=<Frames/>  GraphicType=FromGeometry  MarkerShape=Sphere  MarkerSize=10  MarkerSizeUnits=m  GraphicVisPropType=SimpleVisualProperties  GraphicDiffuseColor=be_color  GraphicSpecularColor=[0.5 0.5 0.5 1.0]  GraphicAmbientColor=[0.15 0.15 0.15 1.0]  GraphicEmissiveColor=[0.0 0.0 0.0 1.0]  GraphicShininess=75  GraphicOpacity=be_opacity  GeometryShape=GeneralExtrusion  RectangleSize=[1 1]  RectangleSizeUnits=m  BrickDimensions=[1 1 1]  BrickDimensionUnits=m  CylinderRadius=1  CylinderRadiusUnits=m  CylinderLength=1  CylinderLengthUnits=m  SphereRadius=1  SphereRadiusUnits=m  EllipsoidRadii=[1 1 1]  EllipsoidRadiiUnits=m  ExtrusionCrossSection=extrusion_data  ExtrusionCrossSectionUnits=m  ExtrusionLength=be_length/2  ExtrusionLengthUnits=m  PolygonNumSides=3  PolygonOuterRadius=1  PolygonOuterRadiusUnits=m  ExtGeomFileType=STL  ExtGeomFileUnits=m  RevolutionCrossSection=[1 1; 1 -1; 2 -1; 2 1]  RevolutionCrossSectionUnits=m  RevolutionExtent=Full  RevolutionAngle=180  RevolutionAngleUnits=deg
  Transform Bending DOF : sm_lib/Frames and Transforms/Rigid Transform  TranslationMethod=StandardAxis  TranslationStandardOffset=be_length/4  TranslationLengthUnit=m  TranslationStandardAxis=+Z  TranslationCartesianOffset=[0 0 0]  TranslationROffset=0  TranslationROffsetUnits=m  TranslationZOffset=0  TranslationZOffsetUnits=m  TranslationThetaOffset=0  TranslationThetaOffsetUnits=deg  RotationMethod=StandardAxis  RotationAngleUnits=deg  RotationStandardAxis=+Y  RotationAngle=90  RotationArbitraryAxis=[0 0 1]  FollAlignAxisA=+X  BaseAlignAxisA=+Y  FollAlignAxisB=+Y  BaseAlignAxisB=+Z  RotationSequenceAxes=FollowerAxes  RotationSequence=XYX  RotationSequenceAngles=[0 0 0]  RotationSequenceAnglesUnits=deg  RotationMatrix=[1 0 0; 0 1 0; 0 0 1]
  Transform HalfBeamB : sm_lib/Frames and Transforms/Rigid Transform  TranslationMethod=StandardAxis  TranslationStandardOffset=be_length/4  TranslationLengthUnit=m  TranslationStandardAxis=+Z  TranslationCartesianOffset=[0 0 0]  TranslationROffset=0  TranslationROffsetUnits=m  TranslationZOffset=0  TranslationZOffsetUnits=m  TranslationThetaOffset=0  TranslationThetaOffsetUnits=deg  RotationMethod=None  RotationAngleUnits=deg  RotationStandardAxis=+Z  RotationAngle=0  RotationArbitraryAxis=[0 0 1]  FollAlignAxisA=+X  BaseAlignAxisA=+Y  FollAlignAxisB=+Y  BaseAlignAxisB=+Z  RotationSequenceAxes=FollowerAxes  RotationSequence=XYX  RotationSequenceAngles=[0 0 0]  RotationSequenceAnglesUnits=deg  RotationMatrix=[1 0 0; 0 1 0; 0 0 1]
  Transform HalfBeamF : sm_lib/Frames and Transforms/Rigid Transform  TranslationMethod=StandardAxis  TranslationStandardOffset=-be_length/4  TranslationLengthUnit=m  TranslationStandardAxis=+Z  TranslationCartesianOffset=[0 0 0]  TranslationROffset=0  TranslationROffsetUnits=m  TranslationZOffset=0  TranslationZOffsetUnits=m  TranslationThetaOffset=0  TranslationThetaOffsetUnits=deg  RotationMethod=StandardAxis  RotationAngleUnits=deg  RotationStandardAxis=+Y  RotationAngle=90  RotationArbitraryAxis=[0 0 1]  FollAlignAxisA=+X  BaseAlignAxisA=+Y  FollAlignAxisB=+Y  BaseAlignAxisB=+Z  RotationSequenceAxes=FollowerAxes  RotationSequence=XYX  RotationSequenceAngles=[0 0 0]  RotationSequenceAnglesUnits=deg  RotationMatrix=[1 0 0; 0 1 0; 0 0 1]
  B : PMIOPort  Port=1  Side=Left
  F : PMIOPort  Port=2  Side=Right
  connections:
  " Transform BeamF"/RConn1 -- F/RConn1
  Transform HalfBeamB/LConn1 -- B/RConn1
  " Transform BeamF"/LConn1 -- Solid HalfBeamF/RConn1 -- Transform HalfBeamF/LConn1
  Transform HalfBeamB/RConn1 -- Solid HalfBeamB/RConn1 -- Transform Bending DOF/LConn1
  Flex Joint/RConn1 -- Transform HalfBeamF/RConn1
  Flex Joint/LConn1 -- Transform Bending DOF/RConn1
